simulink model "Aircraft"  (Simulink 8.7)
settings: Solver=ode45  StartTime=0.0  StopTime=10.0  RelTol=1e-3
values from neighbouring files (symbols this model uses):
  Inertia = [9496,0,982 ... (first row only)    [main.m]
  mass = 636.94    [main.m]
undefined symbols (not defined in the file): alpha, altitude, velocity
libraries: aerolib6dof x4, aerolibobsolete x1, aerolibutil x1, aerolibgravity2 x1
settings Model: Creator=ThinkPad User  LastModifiedBy=Gray
settings DataIOCC: SignalLoggingSaveFormat=ModelDataLogs
settings OptimizationCC: ExpressionDepthLimit=2147483647
settings DebuggingCC: SolverPrmCheckMsg=warning  FcnCallInpInsideContextMsg=EnableAllAsWarning  StateNameClashWarn=warning
settings ConfigComp: CovSFcnEnable=off

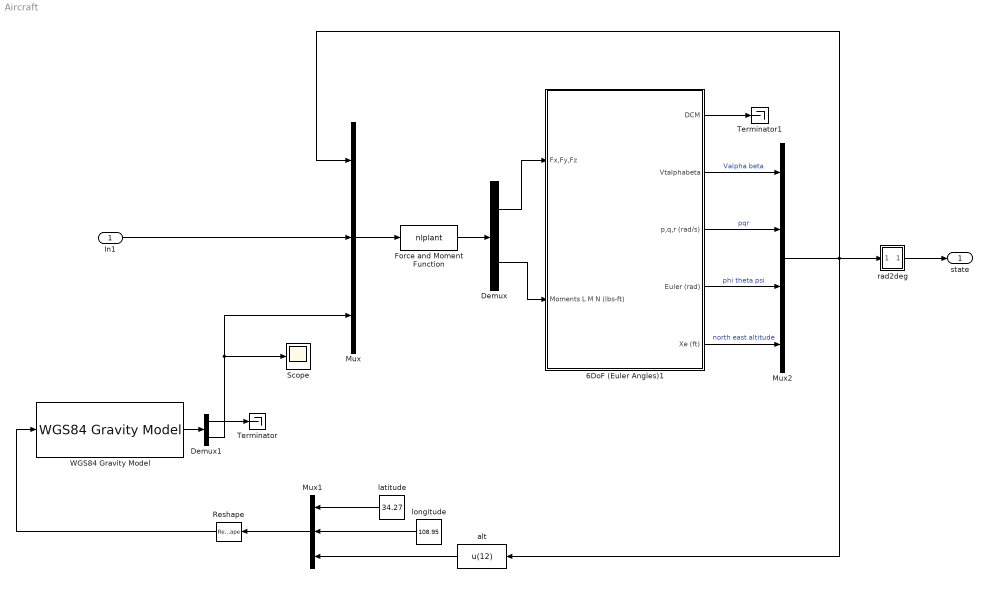
== system Aircraft ==
  In1 : Inport
  6DoF (Euler Angles)1 : Subsystem  RequirementInfo={} %GIDa_d4817105_5849_45f3_a0e7_aea0e0cf3329  AncestorBlock=aerolib6dof/6DoF (Euler Angles)  mask(6DoF (Euler Angles) EoM){xme_0=[0,0,altitude], Vmw_0=[velocity,alpha,0], eul_0=[0 0 0], pm_0=[0 0 0], mass=mass, Inertia=Inertia}
      mask prompts: xme_0 "Initial position in inertial axes [Xe,Ye,Ze] (ft):"; Vmw_0 "Vt  alpha  beta"; eul_0 "Initial Euler orientation [roll, pitch, yaw] (rad):"; pm_0 "Initial body rotation rates [p,q,r] (rad/s):"; mass "Mass (slugs):"; Inertia "Inertia matrix (slugs.ft^2):"
      mask help:
      | Integrate the six-degrees-of-freedom equations of motion using an Euler angle representation for the orientation of the body in space.
      |
      | Inputs are forces on the body in x-axis, y-axis, and z-axis; and moments on the body along x-axis, y-axis, and z-axis. Outputs are translational velocity in x-axis, y-axis, and z-axis in inertial coordinates; position in x-axis, y-axis, and z-axis in inertial coordinates; phi, theta, and psi; 3-by-3 direction cosine matrix; translational velocity in x-axis, y-axis, and z-axis in body coordinates; roll, pitch, and yaw rate; and roll, pitch, and yaw acceleration.
      mask Help: web(asbhelp('6dofeulerangles'));
      mask Display: disp('Euler\nAngles')
  Demux : Demux  Outputs=[3,3]
  Demux1 : Demux  Outputs=2
  Force and Moment Function : MATLABFcn  MATLABFcn=nlplant  OutputDimensions=6
  Mux : Mux  Inputs=[12,4,1]
  Mux1 : Mux  Inputs=3
  Mux2 : Mux
  Reshape : Reshape
  Scope : Scope
  Terminator : Terminator
  Terminator1 : Terminator
  "WGS84 Gravity Model " : aerolibgravity2/WGS84 Gravity Model   model=WGS84 Taylor Series  units=English  no_atmos=on  precessing=on  jd_loc=off  month=October  day=10  year=2004  no_centrifugal=on  action=Warning
  alt : Fcn  Expr=u(12)
  latitude : Constant  Value=34.27
  longitude : Constant  Value=108.95
  rad2deg : Subsystem
  state : Outport
  wires:
  Force and Moment Function/1 -> Demux/1
  Mux/1 -> Force and Moment Function/1
  latitude/1 -> Mux1/1
  longitude/1 -> Mux1/2
  Mux1/1 -> Reshape/1
  Reshape/1 -> "WGS84 Gravity Model "/1
  alt/1 -> Mux1/3
  "WGS84 Gravity Model "/1 -> Demux1/1
  Demux1/2 -> Mux/3, Scope/1
  Demux1/1 -> Terminator/1
  In1/1 -> Mux/2
  Demux/1 -> 6DoF (Euler Angles)1/1(Fx,Fy,Fz)
  Demux/2 -> 6DoF (Euler Angles)1/2(Moments L M N (lbs-ft))
  6DoF (Euler Angles)1/2(Vtalphabeta) -> Mux2/1  "Valpha beta"
  6DoF (Euler Angles)1/3(p,q,r (rad/s)) -> Mux2/2  "pqr"
  6DoF (Euler Angles)1/4(Euler (rad)) -> Mux2/3  "phi theta psi"
  6DoF (Euler Angles)1/5(Xe (ft)) -> Mux2/4  "north east altitude"
  Mux2/1 -> rad2deg/1(In1), alt/1, Mux/1
  6DoF (Euler Angles)1/1(DCM) -> Terminator1/1
  rad2deg/1(Out1) -> state/1

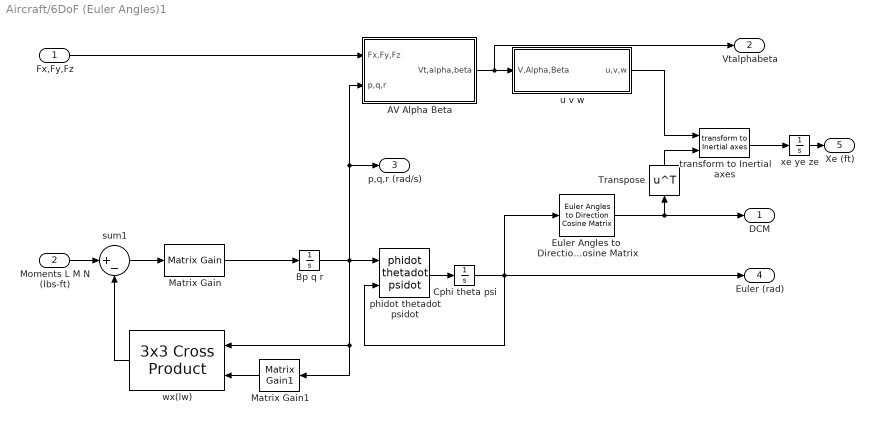
== system Aircraft/6DoF (Euler Angles)1 ==
  Fx,Fy,Fz : Inport  RequirementInfo={} %GIDa_50deebb6_e608_4b93_ae14_8ae4d93d6e74
  Moments L M N (lbs-ft) : Inport  RequirementInfo={} %GIDa_e40f5b11_e422_4137_89eb_88ece0c15722  Port=2
  AV Alpha Beta : Subsystem  RequirementInfo={} %GIDa_eb8f66d3_e87e_40e3_bb04_5553ed292a4e
  Bp q r : Integrator  RequirementInfo={} %GIDa_a671214d_1eac_4e5d_a94c_9b2afa99be54  InitialCondition=pm_0
  Cphi theta psi : Integrator  RequirementInfo={} %GIDa_a2613a5d_07c8_4ac6_b4a2_6282c027a544  InitialCondition=eul_0
  Euler Angles to  Direction Cosine Matrix : aerolibobsolete/Euler Angles to  Direction Cosine Matrix
  Matrix Gain : aerolib6dof/6DoF (Euler Angles)/Matrix Gain  K=inv(Inertia)
  Matrix Gain1 : aerolib6dof/6DoF (Euler Angles)/Matrix Gain1  K=Inertia
  Transpose : Math  RequirementInfo={} %GIDa_4073813e_d529_45cf_b328_16ff15068b63  Operator=transpose  SaturateOnIntegerOverflow=on
  phidot thetadot psidot : aerolib6dof/6DoF (Euler Angles)/phidot thetadot psidot
  sum1 : Sum  RequirementInfo={} %GIDa_5727ba8f_3d30_4102_a894_495d9e941459  Inputs=|+-  SaturateOnIntegerOverflow=on  InputSameDT=on  OutDataTypeStr=Inherit: Same as first input
  "transform to Inertial axes " : aerolib6dof/6DoF (Euler Angles)/transform to Inertial axes   SystemSampleTime=-1
  u v w : Subsystem  RequirementInfo={} %GIDa_34f394f1_1ec2_4d42_a494_c9c240162967
  wx(lw) : aerolibutil/3x3 Cross Product
  xe ye ze : Integrator  RequirementInfo={} %GIDa_103d2c49_44f3_48ac_8ef4_784bc4667605  InitialCondition=xme_0
  DCM : Outport  RequirementInfo={} %GIDa_66647e00_1492_4a29_b65e_3ef278052736
  Vtalphabeta : Outport  RequirementInfo={} %GIDa_461d83bf_0c74_4cec_bcfd_09c1fd0d38d8  Port=2
  p,q,r (rad/s) : Outport  RequirementInfo={} %GIDa_77874acf_9ec3_4049_8483_464677aab7bd  Port=3
  Euler (rad) : Outport  RequirementInfo={} %GIDa_376b897e_78d7_4a98_83d7_1105b162f5de  Port=4
  Xe (ft) : Outport  RequirementInfo={} %GIDa_389fac20_e9e2_45c4_b750_d1db65605663  Port=5
  wires:
  Transpose/1 -> "transform to Inertial axes "/2
  Euler Angles to  Direction Cosine Matrix/1 -> Transpose/1, DCM/1
  Matrix Gain/1 -> Bp q r/1
  wx(lw)/1 -> sum1/2
  Matrix Gain1/1 -> wx(lw)/2
  Moments L M N (lbs-ft)/1 -> sum1/1
  sum1/1 -> Matrix Gain/1
  Bp q r/1 -> Matrix Gain1/1, wx(lw)/1, phidot thetadot psidot/1, p,q,r (rad/s)/1, AV Alpha Beta/2(p,q,r)
  "transform to Inertial axes "/1 -> xe ye ze/1
  xe ye ze/1 -> Xe (ft)/1
  u v w/1(u,v,w) -> "transform to Inertial axes "/1
  Cphi theta psi/1 -> phidot thetadot psidot/2, Euler Angles to  Direction Cosine Matrix/1, Euler (rad)/1
  phidot thetadot psidot/1 -> Cphi theta psi/1
  AV Alpha Beta/1(Vt,alpha,beta) -> Vtalphabeta/1, u v w/1(V,Alpha,Beta)
  Fx,Fy,Fz/1 -> AV Alpha Beta/1(Fx,Fy,Fz)

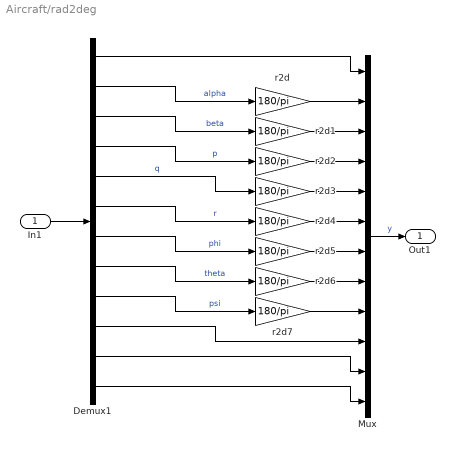
== system Aircraft/rad2deg ==
  In1 : Inport
  Demux1 : Demux  Outputs=12
  Mux : Mux  Inputs=12
  r2d{,1..7} (8 alike) : Gain  Gain=180/pi  SaturateOnIntegerOverflow=on  OutDataTypeStr=Inherit: Same as input  ParamDataTypeStr=Inherit: Same as input
  Out1 : Outport
  wires:
  In1/1 -> Demux1/1
  r2d2/1 -> Mux/4
  r2d1/1 -> Mux/3
  r2d/1 -> Mux/2
  Mux/1 -> Out1/1  "y"
  Demux1/1 -> Mux/1
  Demux1/2 -> r2d/1  "alpha"
  Demux1/3 -> r2d1/1  "beta"
  Demux1/4 -> r2d2/1  "p"
  Demux1/5 -> r2d3/1  "q"
  r2d3/1 -> Mux/5
  r2d4/1 -> Mux/6
  r2d5/1 -> Mux/7
  r2d6/1 -> Mux/8
  r2d7/1 -> Mux/9
  Demux1/6 -> r2d4/1  "r"
  Demux1/7 -> r2d5/1  "phi"
  Demux1/8 -> r2d6/1  "theta"
  Demux1/9 -> r2d7/1  "psi"
  Demux1/10 -> Mux/10
  Demux1/11 -> Mux/11
  Demux1/12 -> Mux/12

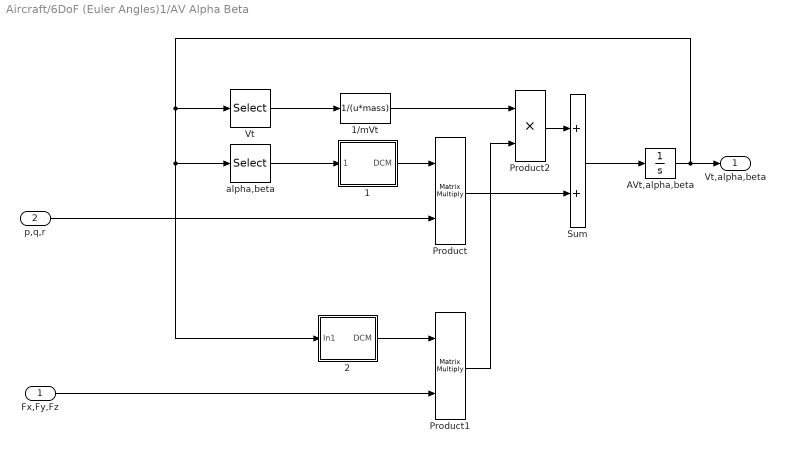
== system Aircraft/6DoF (Euler Angles)1/AV Alpha Beta ==
  Fx,Fy,Fz : Inport  RequirementInfo={} %GIDa_7bb51cb0_3945_46c1_baa0_ab840e9ba37f
  p,q,r : Inport  RequirementInfo={} %GIDa_0cc2a496_759d_4347_9ef1_2d02df0cff82  Port=2
  1 : Subsystem  RequirementInfo={} %GIDa_00e2383c_2bcb_4a06_88cb_7fff4720b52a  AncestorBlock="aerolibtransform/Euler Angles to  Direction Cosine Matrix"  mask(Euler2DCM){}
      mask help: Determine the 3-by-3 direction cosine matrix (DCM) from an Euler orientation (roll, pitch, yaw). The output DCM transforms vectors from inertial axes to body axes.
      mask Help: web(asbhelp('euleranglestodirectioncosinematrix'));
      mask Display: disp('Eul2DCM')
  1/mVt : Fcn  RequirementInfo={} %GIDa_441ee70e_4018_4f67_8b83_522a1466e93a  Expr=1/(u*mass)
  2 : Subsystem  RequirementInfo={} %GIDa_e562dd94_87bd_42c1_8c31_67292e00c26d  AncestorBlock="aerolibtransform/Euler Angles to  Direction Cosine Matrix"  mask(Euler2DCM){}
      mask help: Determine the 3-by-3 direction cosine matrix (DCM) from an Euler orientation (roll, pitch, yaw). The output DCM transforms vectors from inertial axes to body axes.
      mask Help: web(asbhelp('euleranglestodirectioncosinematrix'));
      mask Display: disp('Eul2DCM')
  AVt,alpha,beta : Integrator  RequirementInfo={} %GIDa_4411e8b6_9120_4ab2_83dd_6740a76f6195  InitialCondition=Vmw_0
  Product : Product  RequirementInfo={} %GIDa_bc1df105_bd00_499a_b85f_f50ea7613304  Multiplication=Matrix(*)  SaturateOnIntegerOverflow=on  OutDataTypeStr=Inherit: Same as first input
  Product1 : Product  RequirementInfo={} %GIDa_97231b1f_6e33_4f46_af19_87f640ee8de7  Multiplication=Matrix(*)  SaturateOnIntegerOverflow=on  OutDataTypeStr=Inherit: Same as first input
  Product2 : Product  RequirementInfo={} %GIDa_e6bfeb5d_db89_4775_bb2e_4866f70b0484  SaturateOnIntegerOverflow=on  OutDataTypeStr=Inherit: Same as first input
  Sum : Sum  RequirementInfo={} %GIDa_b83f2482_5786_4159_9686_9019076a89da  SaturateOnIntegerOverflow=on
  Vt : Selector  RequirementInfo={} %GIDa_eb74c3f2_bf81_418c_bcde_5183d768776b  InputPortWidth=3  IndexOptions=Index vector (dialog)  Indices=[1]  OutputSizes=1
  alpha,beta : Selector  RequirementInfo={} %GIDa_b98cd3b4_e809_428b_84ea_ba562b3c178d  InputPortWidth=3  IndexOptions=Index vector (dialog)  Indices=[2 3]  OutputSizes=1
  Vt,alpha,beta : Outport  RequirementInfo={} %GIDa_7cd0454c_7d9f_448a_a3f2_4156dbfeabbb
  wires:
  1/1(DCM) -> Product/1
  p,q,r/1 -> Product/2
  2/1(DCM) -> Product1/1
  alpha,beta/1 -> 1/1(aeodata)
  Fx,Fy,Fz/1 -> Product1/2
  Vt/1 -> 1/mVt/1
  Product1/1 -> Product2/2
  1/mVt/1 -> Product2/1
  Product2/1 -> Sum/1
  Product/1 -> Sum/2
  Sum/1 -> AVt,alpha,beta/1
  AVt,alpha,beta/1 -> Vt,alpha,beta/1, Vt/1, 2/1(In1), alpha,beta/1

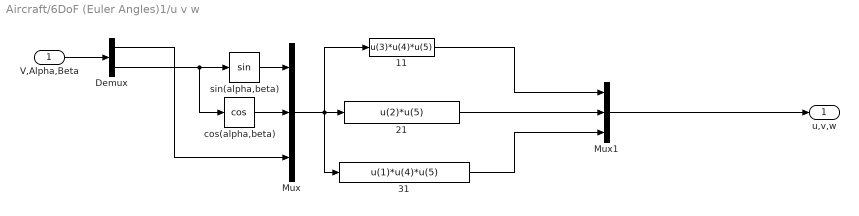
== system Aircraft/6DoF (Euler Angles)1/u v w ==
  V,Alpha,Beta : Inport  RequirementInfo={} %GIDa_bc7ba1e4_ca59_4d4d_9385_e967ef95c45e
  11 : Fcn  RequirementInfo={} %GIDa_d1448c9d_88a7_4c90_83c7_bcba8a811a4b  Expr=u(3)*u(4)*u(5)
  21 : Fcn  RequirementInfo={} %GIDa_585b70a6_50fd_437a_a6ba_b9bf5d6aa185  Expr=u(2)*u(5)
  31 : Fcn  RequirementInfo={} %GIDa_e309239b_cfe3_49a7_b721_357c3c1dd284  Expr=u(1)*u(4)*u(5)
  Demux : Demux  RequirementInfo={} %GIDa_25d931f2_d6b5_4ffe_90b5_d033950a62dc  Outputs=[1,2]
  Mux : Mux  RequirementInfo={} %GIDa_a19af7d9_c990_4521_bb93_a35e8c6a2697  Inputs=3
  Mux1 : Mux  RequirementInfo={} %GIDa_1bf51c2d_67b4_4446_8d56_550fe5a91e21  Inputs=3
  cos(alpha,beta) : Trigonometry  RequirementInfo={} %GIDa_f3a548b7_2684_4854_b70e_b81931377269  Operator=cos
  sin(alpha,beta) : Trigonometry  RequirementInfo={} %GIDa_47f58ccd_2873_4c88_80c3_a04aeb439201
  u,v,w : Outport  RequirementInfo={} %GIDa_61abd662_4a14_4ed2_9676_4f7da0bab78e
  wires:
  V,Alpha,Beta/1 -> Demux/1
  Mux1/1 -> u,v,w/1
  sin(alpha,beta)/1 -> Mux/1
  cos(alpha,beta)/1 -> Mux/2
  Mux/1 -> 11/1, 21/1, 31/1
  Demux/1 -> Mux/3
  11/1 -> Mux1/1
  21/1 -> Mux1/2
  31/1 -> Mux1/3
  Demux/2 -> sin(alpha,beta)/1, cos(alpha,beta)/1

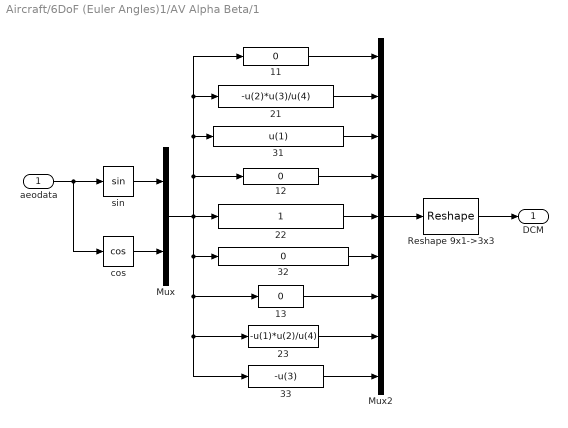
== system Aircraft/6DoF (Euler Angles)1/AV Alpha Beta/1 ==
  aeodata : Inport  RequirementInfo={} %GIDa_ba8e2810_01f1_4fdb_9f21_f0b65585a459
  11 : Fcn  RequirementInfo={} %GIDa_57400c4a_5d2f_4f2c_b9be_52fc91316fa6  Expr=0
  12 : Fcn  RequirementInfo={} %GIDa_075c3dff_44c7_411b_98ef_8ed4f42e0709  Expr=0
  13 : Fcn  RequirementInfo={} %GIDa_9949c464_076c_4477_96bb_f498b18d6943  Expr=0
  21 : Fcn  RequirementInfo={} %GIDa_48ef4c9c_8dda_4009_83e4_2ae5732457a2  Expr=-u(2)*u(3)/u(4)
  22 : Fcn  RequirementInfo={} %GIDa_0d283cdd_be33_410f_804d_3e34f3def749  Expr=1
  23 : Fcn  RequirementInfo={} %GIDa_ad97de75_ba20_497e_b9c0_83ed3ac9c5c5  Expr=-u(1)*u(2)/u(4)
  31 : Fcn  RequirementInfo={} %GIDa_24aabab0_7c41_4ece_8629_78386b8325a1  Expr=u(1)
  32 : Fcn  RequirementInfo={} %GIDa_809f99ec_fa07_4b5d_9dbe_2b96cbc4888b  Expr=0
  33 : Fcn  RequirementInfo={} %GIDa_3743a510_c15c_4b0e_8624_907458b1d3a9  Expr=-u(3)
  Mux : Mux  RequirementInfo={} %GIDa_3eaf6c64_04bc_443d_8925_1d49a11de2f0  Inputs=2
  Mux2 : Mux  RequirementInfo={} %GIDa_411ce7d6_dab1_4a24_9621_dff14cd768c4  Inputs=9
  Reshape 9x1->3x3 : Reshape  RequirementInfo={} %GIDa_1c2de4d1_b8c4_4c5b_afb1_a6f6ac47ba1f  OutputDimensionality=Customize  OutputDimensions=[3,3]
  cos : Trigonometry  RequirementInfo={} %GIDa_79eeb12c_7457_413b_b078_04da64d99113  Operator=cos
  sin : Trigonometry  RequirementInfo={} %GIDa_4a29c1ca_15b3_4fed_96f7_e023182b1369
  DCM : Outport  RequirementInfo={} %GIDa_1485531f_a1a3_4e4d_b063_67817368ac9f  InitialOutput=0
  wires:
  33/1 -> Mux2/9
  23/1 -> Mux2/8
  13/1 -> Mux2/7
  32/1 -> Mux2/6
  22/1 -> Mux2/5
  12/1 -> Mux2/4
  31/1 -> Mux2/3
  21/1 -> Mux2/2
  11/1 -> Mux2/1
  Mux2/1 -> Reshape 9x1->3x3/1
  Reshape 9x1->3x3/1 -> DCM/1
  sin/1 -> Mux/1
  cos/1 -> Mux/2
  aeodata/1 -> sin/1, cos/1
  Mux/1 -> 22/1, 11/1, 21/1, 31/1, 12/1, 32/1, 13/1, 23/1, 33/1

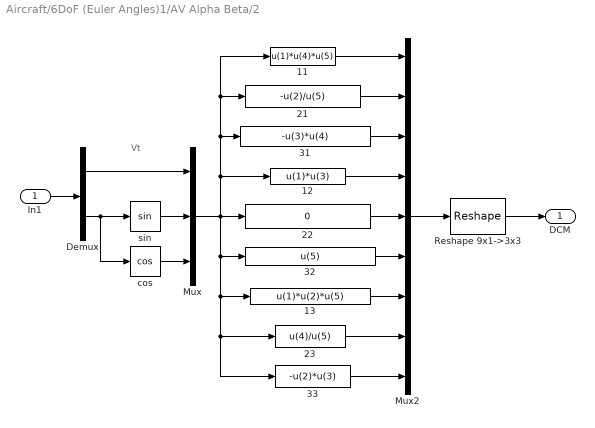
== system Aircraft/6DoF (Euler Angles)1/AV Alpha Beta/2 ==
  note: Vt
  In1 : Inport  RequirementInfo={} %GIDa_a2352181_f5da_4082_bf4e_6ff0f844b052
  11 : Fcn  RequirementInfo={} %GIDa_e34a77d4_6152_4abe_96f7_79c9059a28a3  Expr=u(1)*u(4)*u(5)
  12 : Fcn  RequirementInfo={} %GIDa_e5cb5a61_75f1_4b72_94f6_287430dcc471  Expr=u(1)*u(3)
  13 : Fcn  RequirementInfo={} %GIDa_7bd4546b_c411_4881_b492_c1316203fa4e  Expr=u(1)*u(2)*u(5)
  21 : Fcn  RequirementInfo={} %GIDa_65b9c7ef_9dfb_4d27_b595_8c82be890fce  Expr=-u(2)/u(5)
  22 : Fcn  RequirementInfo={} %GIDa_d5902911_3fb8_4d4e_bb2c_dee27ba265f8  Expr=0
  23 : Fcn  RequirementInfo={} %GIDa_937321a0_3435_470d_88df_6e5b22da0dbb  Expr=u(4)/u(5)
  31 : Fcn  RequirementInfo={} %GIDa_246008ef_721a_4cee_9833_b539ed148a17  Expr=-u(3)*u(4)
  32 : Fcn  RequirementInfo={} %GIDa_dbba2025_0c7a_47b6_904a_d5660c245103  Expr=u(5)
  33 : Fcn  RequirementInfo={} %GIDa_46e45d69_8601_406d_ad3c_263fbfe44c10  Expr=-u(2)*u(3)
  Demux : Demux  RequirementInfo={} %GIDa_4fa5526c_095a_435b_b65d_4820edfb95c4  Outputs=[1 2]
  Mux : Mux  RequirementInfo={} %GIDa_aafe697c_8f9f_49ad_9e49_7374d9b05ccd  Inputs=[1 2 2]
  Mux2 : Mux  RequirementInfo={} %GIDa_f3117a7a_a117_4748_9dc1_721fa7ff80db  Inputs=9
  Reshape 9x1->3x3 : Reshape  RequirementInfo={} %GIDa_0559aede_13b1_4ce0_9792_17aee6c33006  OutputDimensionality=Customize  OutputDimensions=[3,3]
  cos : Trigonometry  RequirementInfo={} %GIDa_cc95633a_6db8_4bea_89bd_4e34ee23099f  Operator=cos
  sin : Trigonometry  RequirementInfo={} %GIDa_835238d6_62f2_4007_ba6b_23e946efadc1
  DCM : Outport  RequirementInfo={} %GIDa_0fcfee52_9e19_4020_b5a4_203cae3dd876  InitialOutput=0
  wires:
  Mux/1 -> 33/1, 23/1, 13/1, 32/1, 12/1, 31/1, 21/1, 11/1, 22/1
  Demux/2 -> cos/1, sin/1
  Reshape 9x1->3x3/1 -> DCM/1
  Mux2/1 -> Reshape 9x1->3x3/1
  11/1 -> Mux2/1
  21/1 -> Mux2/2
  31/1 -> Mux2/3
  12/1 -> Mux2/4
  22/1 -> Mux2/5
  32/1 -> Mux2/6
  13/1 -> Mux2/7
  23/1 -> Mux2/8
  33/1 -> Mux2/9
  sin/1 -> Mux/2
  cos/1 -> Mux/3
  Demux/1 -> Mux/1
  In1/1 -> Demux/1
